simulink model "FourPidTest"  (R2016a)
settings: Solver=FixedStepAuto  StartTime=0.0  StopTime=10.0  FixedStep=0.002  RelTol=1e-3
libraries: simulink x1
settings Model: Creator=Shinelon  LastModifiedBy=Shinelon

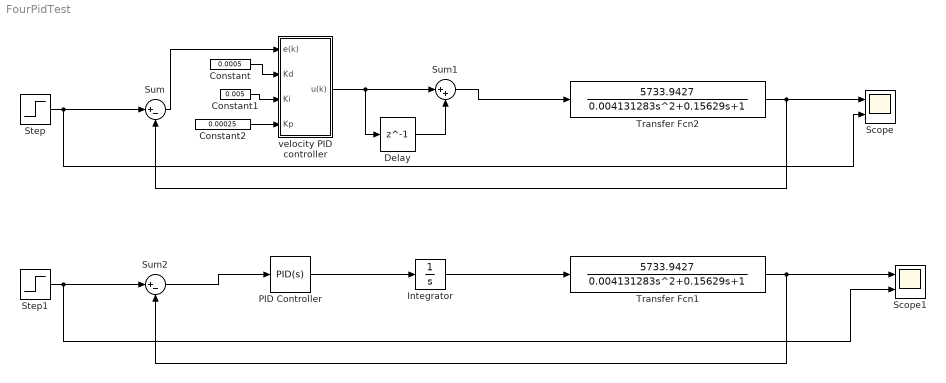
== system FourPidTest ==
  Constant : Constant  Value=0.0005
  Constant1 : Constant  Value=0.005
  Constant2 : Constant  Value=0.00025
  Delay : Delay  DelayLength=1  InitialCondition=0
  Integrator : Integrator
  PID Controller : simulink/Continuous/PID Controller  Controller=PID  TimeDomain=Continuous-time  SampleTime=-1  IntegratorMethod=Forward Euler  FilterMethod=Forward Euler  Form=Parallel  UseFilter=on  ControllerParametersSource=internal  P=0.00030  I=0  D=0.000005  N=2082.18646566435  InitialConditionSource=internal  InitialConditionForIntegrator=0  InitialConditionForFilter=0  ExternalReset=none  LimitOutput=off  UpperSaturationLimit=inf  LowerSaturationLimit=-inf  LinearizeAsGain=on  AntiWindupMode=none  Kb=1  TrackingMode=off  Kt=1  PParamMin=[]  PParamMax=[]  IParamMin=[]  IParamMax=[]  DParamMin=[]  DParamMax=[]  NParamMin=[]  NParamMax=[]  KbParamMin=[]  KbParamMax=[]  KtParamMin=[]  KtParamMax=[]  POutMin=[]  POutMax=[]  IOutMin=[]  IOutMax=[]  DOutMin=[]  DOutMax=[]  NOutMin=[]  NOutMax=[]  KbOutMin=[]  KbOutMax=[]  KtOutMin=[]  KtOutMax=[]  IntegratorOutMin=[]  IntegratorOutMax=[]  FilterOutMin=[]  FilterOutMax=[]  SumOutMin=[]  SumOutMax=[]  SumI1OutMin=[]  SumI1OutMax=[]  SumI2OutMin=[]  SumI2OutMax=[]  SumI3OutMin=[]  SumI3OutMax=[]  SumDOutMin=[]  SumDOutMax=[]  SaturationOutMin=[]  SaturationOutMax=[]  IntegratorContinuousStateAttributes=''  IntegratorStateMustResolveToSignalObject=off  IntegratorRTWStateStorageClass=Auto  FilterContinuousStateAttributes=''  FilterStateMustResolveToSignalObject=off  FilterRTWStateStorageClass=Auto  DifferentiatorICPrevScaledInput=0  DifferentiatorOutMin=[]  DifferentiatorOutMax=[]
  Scope : Scope  NumInputPorts=2
  Scope1 : Scope  NumInputPorts=2
  Step : Step  SampleTime=0
  Step1 : Step  SampleTime=0
  Sum : Sum  Inputs=|+-
  Sum1 : Sum  Inputs=|++
  Sum2 : Sum  Inputs=|+-
  Transfer Fcn1 : TransferFcn  Numerator=[5733.9427]  Denominator="[0.004131283  0.15629 1]"
  Transfer Fcn2 : TransferFcn  Numerator=[5733.9427]  Denominator="[0.004131283  0.15629 1]"
  "velocity PID controller " : Subsystem
  wires:
  Step/1 -> Scope/2, Sum/1
  Transfer Fcn2/1 -> Sum/2, Scope/1
  Constant/1 -> "velocity PID controller "/2("Kd ")
  Constant1/1 -> "velocity PID controller "/3("Ki ")
  Constant2/1 -> "velocity PID controller "/4("Kp ")
  Sum/1 -> "velocity PID controller "/1(e(k))
  "velocity PID controller "/1(u(k)) -> Delay/1, Sum1/1
  Sum1/1 -> Transfer Fcn2/1
  Delay/1 -> Sum1/2
  Step1/1 -> Scope1/2, Sum2/1
  Transfer Fcn1/1 -> Sum2/2, Scope1/1
  Sum2/1 -> PID Controller/1
  Integrator/1 -> Transfer Fcn1/1
  PID Controller/1 -> Integrator/1

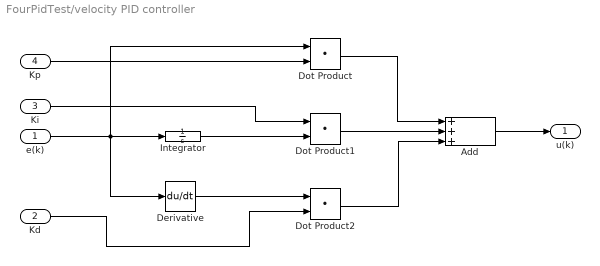
== system FourPidTest/velocity PID controller  ==
  e(k) : Inport
  "Kd " : Inport  Port=2
  "Ki " : Inport  Port=3
  "Kp " : Inport  Port=4
  Add : Sum  Inputs=+++
  Derivative : Derivative
  Dot Product : DotProduct  InputSameDT=on  OutDataTypeStr=Inherit: Inherit via internal rule
  Dot Product1 : DotProduct  InputSameDT=on  OutDataTypeStr=Inherit: Inherit via internal rule
  Dot Product2 : DotProduct  InputSameDT=on  OutDataTypeStr=Inherit: Inherit via internal rule
  Integrator : Integrator
  u(k) : Outport
  wires:
  "Ki "/1 -> Dot Product1/1
  "Kp "/1 -> Dot Product/2
  Add/1 -> u(k)/1
  Derivative/1 -> Dot Product2/1
  Dot Product/1 -> Add/1
  Dot Product2/1 -> Add/3
  Integrator/1 -> Dot Product1/2
  "Kd "/1 -> Dot Product2/2
  Dot Product1/1 -> Add/2
  e(k)/1 -> Dot Product/1, Integrator/1, Derivative/1
